simulink model "MovingAvg5"  (R2022a)
settings: Solver=FixedStepAuto  StartTime=0.0  StopTime=2500  FixedStep=1/3600  RelTol=1e-3
undefined symbols (not defined in the file or in its folder): dspblkCoreblockFVToolHelper, gcbh, sigbuilder_block
settings Model: SimulationMode=accelerator  Creator=rupak  LastModifiedBy=rupak
settings ConfigComp: DVTestSuiteOptimization=Auto  DVDefectChecker=off  DVDetectOutOfBounds=on  DVModelReferenceHarness=on  DVHarnessSource=Signal Editor

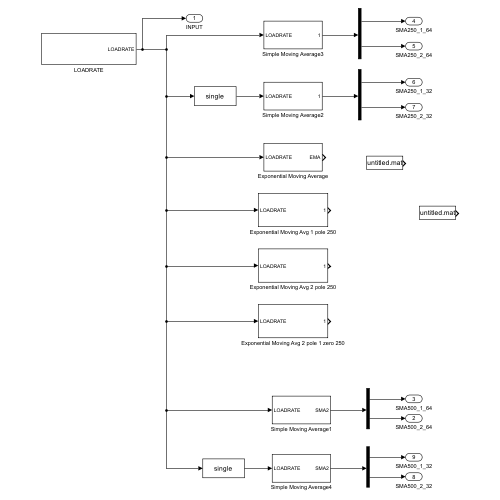
[thumbnail: Simulink's stored preview of the top-level diagram]
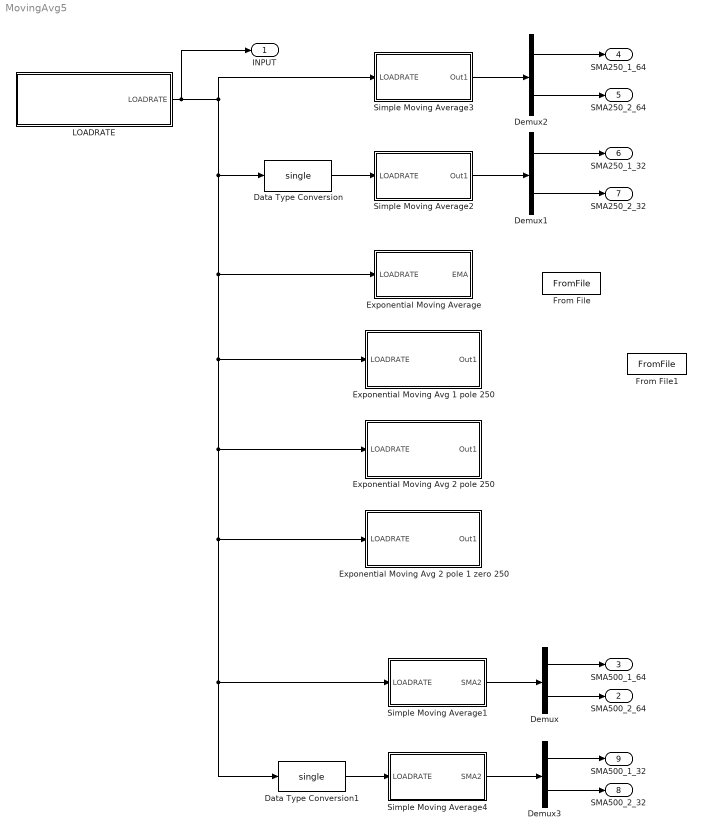
== system MovingAvg5 ==
  Data Type Conversion : DataTypeConversion  OutDataTypeStr=single  SaturateOnIntegerOverflow=off  RndMeth=Floor
  Data Type Conversion1 : DataTypeConversion  OutDataTypeStr=single  SaturateOnIntegerOverflow=off  RndMeth=Floor
  Demux{,1..3} (4 alike) : Demux  Outputs=2
  Exponential Moving Average : Subsystem
  Exponential Moving Avg 1 pole 250 : Subsystem
  Exponential Moving Avg 2 pole 1 zero 250 : Subsystem
  Exponential Moving Avg 2 pole 250 : Subsystem
  From File : FromFile  SampleTime=0
  From File1 : FromFile  SampleTime=0
  LOADRATE : Subsystem
  Simple Moving Average1 : Subsystem
  Simple Moving Average2 : Subsystem
  Simple Moving Average3 : Subsystem
  Simple Moving Average4 : Subsystem
  INPUT : Outport
  SMA500_2_64 : Outport  Port=2
  SMA500_1_64 : Outport  Port=3
  SMA250_1_64 : Outport  Port=4
  SMA250_2_64 : Outport  Port=5
  SMA250_1_32 : Outport  Port=6
  SMA250_2_32 : Outport  Port=7
  SMA500_2_32 : Outport  Port=8
  SMA500_1_32 : Outport  Port=9
  wires:
  Simple Moving Average1/1(SMA2) -> Demux/1
  Demux/1 -> SMA500_1_64/1
  Demux/2 -> SMA500_2_64/1
  Demux2/2 -> SMA250_2_64/1
  Demux2/1 -> SMA250_1_64/1
  Simple Moving Average3/1(Out1) -> Demux2/1
  LOADRATE/1(LOADRATE) -> Data Type Conversion/1, Exponential Moving Avg 1 pole 250/1(LOADRATE), Exponential Moving Avg 2 pole 250/1(LOADRATE), Exponential Moving Avg 2 pole 1 zero 250/1(LOADRATE), Simple Moving Average1/1(LOADRATE), Data Type Conversion1/1, Exponential Moving Average/1(LOADRATE), Simple Moving Average3/1(LOADRATE), INPUT/1
  Simple Moving Average2/1(Out1) -> Demux1/1
  Demux1/1 -> SMA250_1_32/1
  Demux1/2 -> SMA250_2_32/1
  Demux3/2 -> SMA500_2_32/1
  Demux3/1 -> SMA500_1_32/1
  Simple Moving Average4/1(SMA2) -> Demux3/1
  Data Type Conversion/1 -> Simple Moving Average2/1(LOADRATE)
  Data Type Conversion1/1 -> Simple Moving Average4/1(LOADRATE)

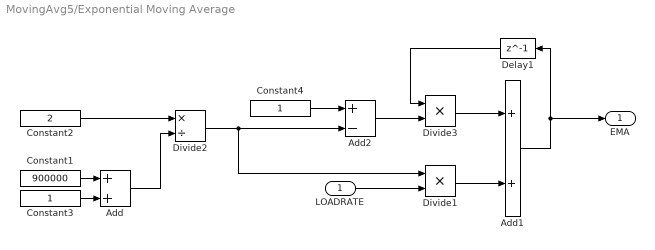
== system MovingAvg5/Exponential Moving Average ==
  LOADRATE : Inport
  Add : Sum
  Add1 : Sum
  Add2 : Sum  Inputs=+-
  Constant1 : Constant  Value=900000  OutDataTypeStr=single
  Constant2 : Constant  Value=2  OutDataTypeStr=single
  Constant3 : Constant  OutDataTypeStr=single
  Constant4 : Constant  OutDataTypeStr=single
  Delay1 : Delay  DelayLength=1  InitialCondition=60
  Divide1 : Product  Inputs=**
  Divide2 : Product  Inputs=*/
  Divide3 : Product  Inputs=**
  EMA : Outport
  wires:
  Add1/1 -> EMA/1, Delay1/1
  Divide1/1 -> Add1/2
  Constant2/1 -> Divide2/1
  Constant1/1 -> Add/1
  Constant3/1 -> Add/2
  Add/1 -> Divide2/2
  Delay1/1 -> Divide3/1
  Divide3/1 -> Add1/1
  Add2/1 -> Divide3/2
  Constant4/1 -> Add2/1
  Divide2/1 -> Add2/2, Divide1/1
  LOADRATE/1 -> Divide1/2

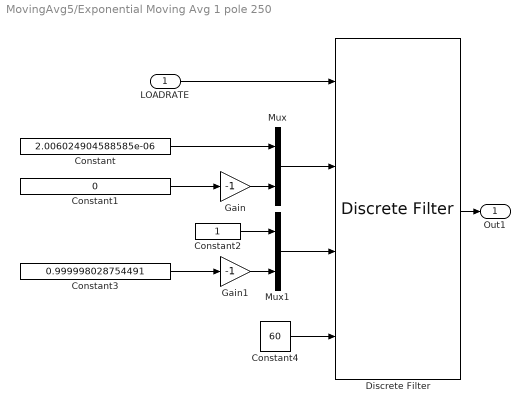
== system MovingAvg5/Exponential Moving Avg 1 pole 250 ==
  LOADRATE : Inport
  Constant : Constant  Value=2.006024904588585e-06
  Constant1 : Constant  Value=0
  Constant2 : Constant
  Constant3 : Constant  Value=0.999998028754491
  Constant4 : Constant  Value=60
  Discrete Filter : DiscreteFilter  LoadFcn=dspblkCoreblockFVToolHelper(gcbh,'load');  NumeratorSource=Input port  DenominatorSource=Input port  InitialStatesSource=Input port  FilterStructure=Direct form II transposed  a0EqualsOne=on
      settings: CopyFcn=dspblkCoreblockFVToolHelper(gcbh,'copy');  DeleteFcn=dspblkCoreblockFVToolHelper(gcbh,'close');  ModelCloseFcn=dspblkCoreblockFVToolHelper(gcbh,'close');  PreSaveFcn=dspblkCoreblockFVToolHelper(gcbh,'presave');  PostSaveFcn=dspblkCoreblockFVToolHelper(gcbh,'postsave');  CloseFcn=dspblkCoreblockFVToolHelper(gcbh,'close');  InputPortMap=u0,p1,p3,p5
  Gain : Gain  Gain=-1
  Gain1 : Gain  Gain=-1
  Mux : Mux  Inputs=2
  Mux1 : Mux  Inputs=2
  Out1 : Outport
  wires:
  Constant4/1 -> Discrete Filter/4
  Constant2/1 -> Mux1/1
  Constant3/1 -> Gain1/1
  Gain1/1 -> Mux1/2
  Mux/1 -> Discrete Filter/2
  Mux1/1 -> Discrete Filter/3
  Constant/1 -> Mux/1
  Constant1/1 -> Gain/1
  Gain/1 -> Mux/2
  LOADRATE/1 -> Discrete Filter/1
  Discrete Filter/1 -> Out1/1

== system MovingAvg5/Exponential Moving Avg 2 pole 1 zero 250 ==
  LOADRATE : Inport
  1st Filt : Subsystem
  2nd Filt : Subsystem
  Out1 : Outport
  wires:
  2nd Filt/1(Out1) -> Out1/1
  1st Filt/1(Out1) -> 2nd Filt/1(In1)
  LOADRATE/1 -> 1st Filt/1(In1)

== system MovingAvg5/Exponential Moving Avg 2 pole 250 ==
  LOADRATE : Inport
  1st Filt : Subsystem
  2nd Filt : Subsystem
  Out1 : Outport
  wires:
  LOADRATE/1 -> 1st Filt/1(In1)
  1st Filt/1(Out1) -> 2nd Filt/1(In1)
  2nd Filt/1(Out1) -> Out1/1

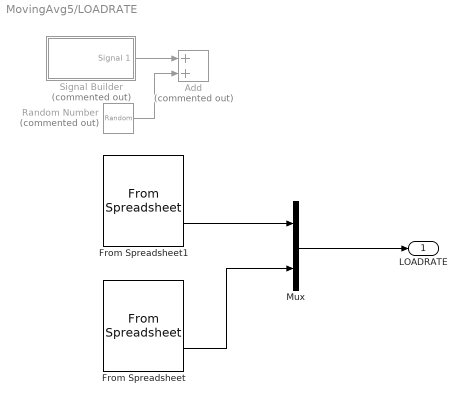
== system MovingAvg5/LOADRATE ==
  Add : Sum  Commented=on
  From Spreadsheet : FromSpreadsheet  FileName=C:\Users\rupak\OneDrive\Documents\MATLAB\Filter\Ransomes_NRTC-Full.xlsx  TreatFirstColumnAs=Data  SampleTime=1/3600
  From Spreadsheet1 : FromSpreadsheet  FileName=C:\Users\rupak\OneDrive\Documents\MATLAB\Filter\NRTC_3.xlsx  SheetName=NRTC_3  OutDataTypeStr=double  TreatFirstColumnAs=Data  SampleTime=1/3600
  Mux : Mux  Inputs=2
  Random Number : RandomNumber  Commented=on  Mean=5  SampleTime=1/3600
  Signal Builder : Subsystem  Tag=STV Subsys  Commented=on  LoadFcn=sigbuilder_block('load');  StartFcn=sigbuilder_block('start');  StopFcn=sigbuilder_block('stop');  ClipboardFcn=sigbuilder_block('clipboard');  mask(Sigbuilder block){tuvar=[0:10]}
      mask help: Simulink:masks:SigbuilderBlock_MD
      mask init:
      | if ~strcmp(get_param(bdroot(gcbh),'SimulationStatus'),'stopped') tuvar = sigbuilder_block('maskInit'); end
      settings: CopyFcn=sigbuilder_block('copy');  DeleteFcn=sigbuilder_block('delete');  ModelCloseFcn=sigbuilder_block('modelClose');  PreSaveFcn=sigbuilder_block('preSave');  PauseFcn=sigbuilder_block('pause');  ContinueFcn=sigbuilder_block('continue');  NameChangeFcn=sigbuilder_block('namechange');  OpenFcn=sigbuilder_block('open',[6 36 1428 675.75 ]);  CloseFcn=sigbuilder_block('close');
      mask Display: plot(0, 0, 100, 100,[2, 2, 32, 32, 2], [68, 8, 8, 68, 68],[32, 2], [38, 38], [32, 19, 2],[53, 60, 44], [32, 17, 17, 2],[16, 16, 31, 31]);txt = getActiveGroup(gcbh);text(2, 100, txt,'verticalAlignment', 'top');
  LOADRATE : Outport  SampleTime=1/3600  LockScale=on
  wires:
  Random Number/1 -> Add/2
  Signal Builder/1(Signal 1) -> Add/1
  Mux/1 -> LOADRATE/1
  From Spreadsheet/2 -> Mux/2
  From Spreadsheet1/2 -> Mux/1

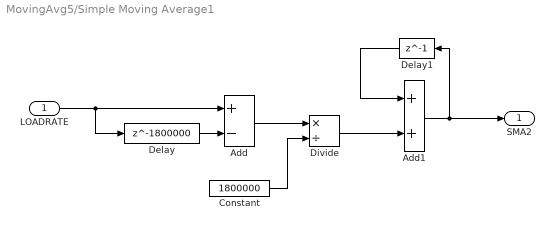
== system MovingAvg5/Simple Moving Average1 ==
  LOADRATE : Inport
  Add : Sum  Inputs=+-
  Add1 : Sum
  Constant : Constant  Value=1800000  OutDataTypeStr=single
  Delay : Delay  DelayLength=1800000  InitialCondition=60
  Delay1 : Delay  DelayLength=1  InitialCondition=60
  Divide : Product  Inputs=*/
  SMA2 : Outport
  wires:
  Divide/1 -> Add1/2
  Add1/1 -> Delay1/1, SMA2/1
  Add/1 -> Divide/1
  LOADRATE/1 -> Add/1, Delay/1
  Constant/1 -> Divide/2
  Delay1/1 -> Add1/1
  Delay/1 -> Add/2

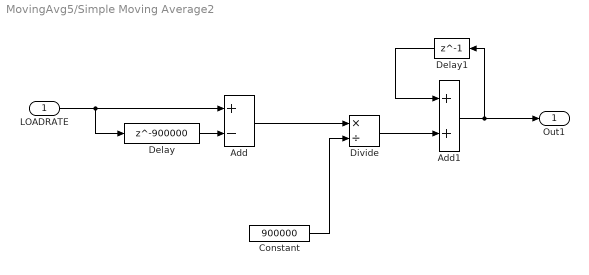
== system MovingAvg5/Simple Moving Average2 ==
  LOADRATE : Inport
  Add : Sum  Inputs=+-
  Add1 : Sum
  Constant : Constant  Value=900000  OutDataTypeStr=Inherit: Inherit via back propagation
  Delay : Delay  DelayLength=900000  InitialCondition=60
  Delay1 : Delay  DelayLength=1  InitialCondition=60
  Divide : Product  Inputs=*/
  Out1 : Outport
  wires:
  Add/1 -> Divide/1
  Delay/1 -> Add/2
  Delay1/1 -> Add1/1
  Constant/1 -> Divide/2
  LOADRATE/1 -> Delay/1, Add/1
  Add1/1 -> Out1/1, Delay1/1
  Divide/1 -> Add1/2

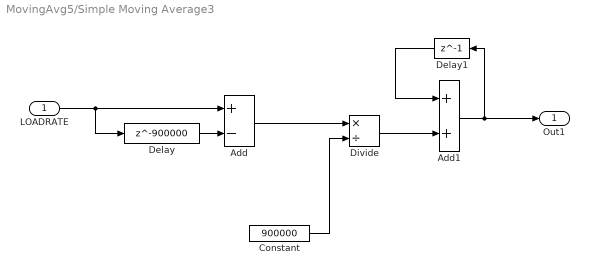
== system MovingAvg5/Simple Moving Average3 ==
  LOADRATE : Inport
  Add : Sum  Inputs=+-
  Add1 : Sum
  Constant : Constant  Value=900000  OutDataTypeStr=Inherit: Inherit via back propagation
  Delay : Delay  DelayLength=900000  InitialCondition=60
  Delay1 : Delay  DelayLength=1  InitialCondition=60
  Divide : Product  Inputs=*/
  Out1 : Outport
  wires:
  Divide/1 -> Add1/2
  Add1/1 -> Delay1/1, Out1/1
  LOADRATE/1 -> Add/1, Delay/1
  Constant/1 -> Divide/2
  Delay1/1 -> Add1/1
  Delay/1 -> Add/2
  Add/1 -> Divide/1

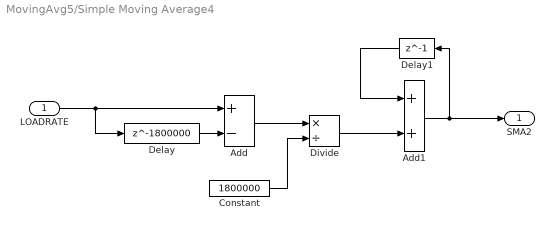
== system MovingAvg5/Simple Moving Average4 ==
  LOADRATE : Inport
  Add : Sum  Inputs=+-
  Add1 : Sum
  Constant : Constant  Value=1800000  OutDataTypeStr=single
  Delay : Delay  DelayLength=1800000  InitialCondition=60
  Delay1 : Delay  DelayLength=1  InitialCondition=60
  Divide : Product  Inputs=*/
  SMA2 : Outport
  wires:
  Delay/1 -> Add/2
  Delay1/1 -> Add1/1
  Constant/1 -> Divide/2
  LOADRATE/1 -> Delay/1, Add/1
  Add/1 -> Divide/1
  Add1/1 -> SMA2/1, Delay1/1
  Divide/1 -> Add1/2

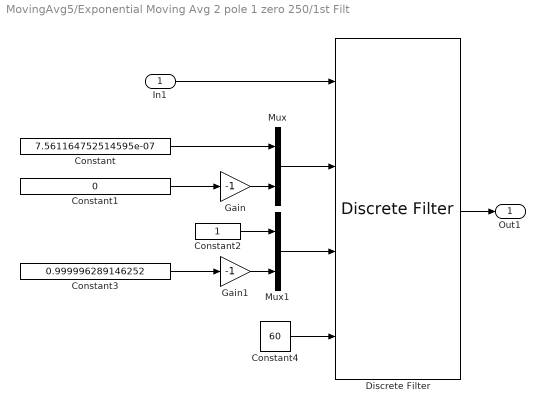
== system MovingAvg5/Exponential Moving Avg 2 pole 1 zero 250/1st Filt ==
  In1 : Inport
  Constant : Constant  Value=7.561164752514595e-07
  Constant1 : Constant  Value=0
  Constant2 : Constant
  Constant3 : Constant  Value=0.999996289146252
  Constant4 : Constant  Value=60
  Discrete Filter : DiscreteFilter  LoadFcn=dspblkCoreblockFVToolHelper(gcbh,'load');  NumeratorSource=Input port  DenominatorSource=Input port  InitialStatesSource=Input port  FilterStructure=Direct form II transposed  a0EqualsOne=on
      settings: CopyFcn=dspblkCoreblockFVToolHelper(gcbh,'copy');  DeleteFcn=dspblkCoreblockFVToolHelper(gcbh,'close');  ModelCloseFcn=dspblkCoreblockFVToolHelper(gcbh,'close');  PreSaveFcn=dspblkCoreblockFVToolHelper(gcbh,'presave');  PostSaveFcn=dspblkCoreblockFVToolHelper(gcbh,'postsave');  CloseFcn=dspblkCoreblockFVToolHelper(gcbh,'close');  InputPortMap=u0,p1,p3,p5
  Gain : Gain  Gain=-1
  Gain1 : Gain  Gain=-1
  Mux : Mux  Inputs=2
  Mux1 : Mux  Inputs=2
  Out1 : Outport
  wires:
  Discrete Filter/1 -> Out1/1
  Constant2/1 -> Mux1/1
  Constant3/1 -> Gain1/1
  Constant1/1 -> Gain/1
  Gain1/1 -> Mux1/2
  Constant4/1 -> Discrete Filter/4
  Constant/1 -> Mux/1
  Gain/1 -> Mux/2
  In1/1 -> Discrete Filter/1
  Mux1/1 -> Discrete Filter/3
  Mux/1 -> Discrete Filter/2

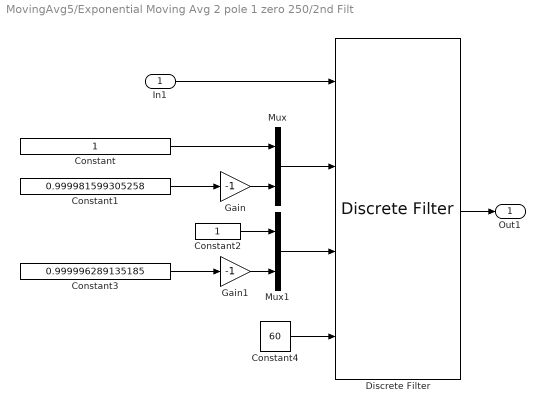
== system MovingAvg5/Exponential Moving Avg 2 pole 1 zero 250/2nd Filt ==
  In1 : Inport
  Constant : Constant
  Constant1 : Constant  Value=0.999981599305258
  Constant2 : Constant
  Constant3 : Constant  Value=0.999996289135185
  Constant4 : Constant  Value=60
  Discrete Filter : DiscreteFilter  LoadFcn=dspblkCoreblockFVToolHelper(gcbh,'load');  NumeratorSource=Input port  DenominatorSource=Input port  InitialStatesSource=Input port  FilterStructure=Direct form II transposed  a0EqualsOne=on
      settings: CopyFcn=dspblkCoreblockFVToolHelper(gcbh,'copy');  DeleteFcn=dspblkCoreblockFVToolHelper(gcbh,'close');  ModelCloseFcn=dspblkCoreblockFVToolHelper(gcbh,'close');  PreSaveFcn=dspblkCoreblockFVToolHelper(gcbh,'presave');  PostSaveFcn=dspblkCoreblockFVToolHelper(gcbh,'postsave');  CloseFcn=dspblkCoreblockFVToolHelper(gcbh,'close');  InputPortMap=u0,p1,p3,p5
  Gain : Gain  Gain=-1
  Gain1 : Gain  Gain=-1
  Mux : Mux  Inputs=2
  Mux1 : Mux  Inputs=2
  Out1 : Outport
  wires:
  Mux/1 -> Discrete Filter/2
  Mux1/1 -> Discrete Filter/3
  In1/1 -> Discrete Filter/1
  Gain/1 -> Mux/2
  Constant/1 -> Mux/1
  Constant4/1 -> Discrete Filter/4
  Gain1/1 -> Mux1/2
  Constant1/1 -> Gain/1
  Constant3/1 -> Gain1/1
  Constant2/1 -> Mux1/1
  Discrete Filter/1 -> Out1/1

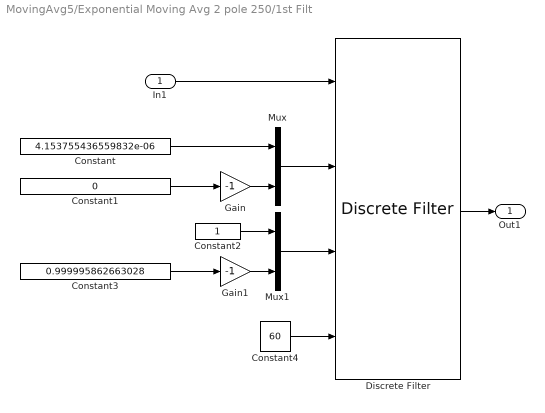
== system MovingAvg5/Exponential Moving Avg 2 pole 250/1st Filt ==
  In1 : Inport
  Constant : Constant  Value=4.153755436559832e-06
  Constant1 : Constant  Value=0
  Constant2 : Constant
  Constant3 : Constant  Value=0.999995862663028
  Constant4 : Constant  Value=60
  Discrete Filter : DiscreteFilter  LoadFcn=dspblkCoreblockFVToolHelper(gcbh,'load');  NumeratorSource=Input port  DenominatorSource=Input port  InitialStatesSource=Input port  FilterStructure=Direct form II transposed  a0EqualsOne=on
      settings: CopyFcn=dspblkCoreblockFVToolHelper(gcbh,'copy');  DeleteFcn=dspblkCoreblockFVToolHelper(gcbh,'close');  ModelCloseFcn=dspblkCoreblockFVToolHelper(gcbh,'close');  PreSaveFcn=dspblkCoreblockFVToolHelper(gcbh,'presave');  PostSaveFcn=dspblkCoreblockFVToolHelper(gcbh,'postsave');  CloseFcn=dspblkCoreblockFVToolHelper(gcbh,'close');  InputPortMap=u0,p1,p3,p5
  Gain : Gain  Gain=-1
  Gain1 : Gain  Gain=-1
  Mux : Mux  Inputs=2
  Mux1 : Mux  Inputs=2
  Out1 : Outport
  wires:
  Mux/1 -> Discrete Filter/2
  Mux1/1 -> Discrete Filter/3
  In1/1 -> Discrete Filter/1
  Gain/1 -> Mux/2
  Constant/1 -> Mux/1
  Constant4/1 -> Discrete Filter/4
  Gain1/1 -> Mux1/2
  Constant1/1 -> Gain/1
  Constant3/1 -> Gain1/1
  Constant2/1 -> Mux1/1
  Discrete Filter/1 -> Out1/1

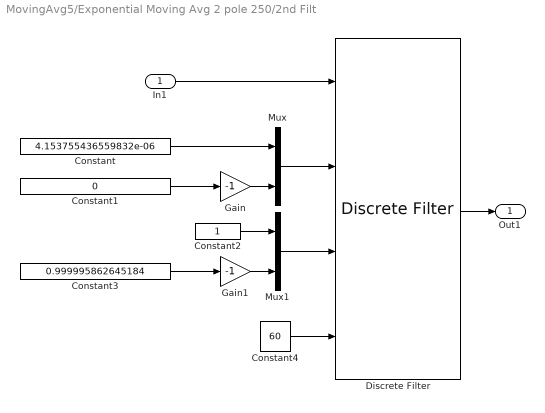
== system MovingAvg5/Exponential Moving Avg 2 pole 250/2nd Filt ==
  In1 : Inport
  Constant : Constant  Value=4.153755436559832e-06
  Constant1 : Constant  Value=0
  Constant2 : Constant
  Constant3 : Constant  Value=0.999995862645184
  Constant4 : Constant  Value=60
  Discrete Filter : DiscreteFilter  LoadFcn=dspblkCoreblockFVToolHelper(gcbh,'load');  NumeratorSource=Input port  DenominatorSource=Input port  InitialStatesSource=Input port  FilterStructure=Direct form II transposed  a0EqualsOne=on
      settings: CopyFcn=dspblkCoreblockFVToolHelper(gcbh,'copy');  DeleteFcn=dspblkCoreblockFVToolHelper(gcbh,'close');  ModelCloseFcn=dspblkCoreblockFVToolHelper(gcbh,'close');  PreSaveFcn=dspblkCoreblockFVToolHelper(gcbh,'presave');  PostSaveFcn=dspblkCoreblockFVToolHelper(gcbh,'postsave');  CloseFcn=dspblkCoreblockFVToolHelper(gcbh,'close');  InputPortMap=u0,p1,p3,p5
  Gain : Gain  Gain=-1
  Gain1 : Gain  Gain=-1
  Mux : Mux  Inputs=2
  Mux1 : Mux  Inputs=2
  Out1 : Outport
  wires:
  Discrete Filter/1 -> Out1/1
  Constant2/1 -> Mux1/1
  Constant3/1 -> Gain1/1
  Constant1/1 -> Gain/1
  Gain1/1 -> Mux1/2
  Constant4/1 -> Discrete Filter/4
  Constant/1 -> Mux/1
  Gain/1 -> Mux/2
  In1/1 -> Discrete Filter/1
  Mux1/1 -> Discrete Filter/3
  Mux/1 -> Discrete Filter/2

== system MovingAvg5/LOADRATE/Signal Builder ==
  Demux : Demux  Tag=STV Demux  Outputs=1
      settings: DisplayOption=none
  FromWs : FromWorkspace  Tag=STV FromWs  VariableName=tuvar
      SigBuilderData=|
      | common.afterFinalStr = 'Extrapolate'
      | common.sampleTime = 0
      | dataSet.timeRange = [0 1500]
      | dataSet.name = 'Group 1'
      | sbobj.Groups.Name = 'Group 1'
      | sbobj.Groups.Signals.Name = 'Signal 1'
      | sbobj.Groups.Signals.XData = [0 4 4 10 12 16 18 20 24 30 36 40 44 50 56 60 60 64 64 70 74 78 80 82 86 88 88 90 92 98 104 108 112 118 122 128 132 138 144 150 154 158 160 162 166 170 174 176 180 182 184 190 196 200 202 208 216 226 232 240 250 260 266 278 284 292 296 300 304 310 316 322 326 338 346 356 362 368 374 378 384 392 400 406 414 420 424 430 432 438 442 446 450 458 464 470 476 482 487 489 490 496 500 508 518 528 536 546 552 558 562 570 582 588 592 598 606 620 626 634 644 650 664 673 674 682 696 706 716 724 734 744 756 764 772 780 790 800 808 816 826 834 844 856 864 872 880 890 904 914 928 942 952 960 972 994 1072 1116 1126 1134 1142 1156 1160 1166 1176 1182 1190 1198 1208 1220 1228 1235 1246 1258 1265 1277 1287 1297 1308 1323 1332 1342 1347 1355 1361 1371 1379 1389 1402 1408 1415 1422 1435 1439 1446 1453 1469 1475 1485 1492 1495 1500]
      | sbobj.Groups.Signals.YData = [2 96.2 69.2 84 75 56.8 90 74.4 80.8 65.2 91 85.4 67.4 77.4 55.6 61 48 18.6 31.6 51.4 51.4 38.4 56.4 63.4 86.6 78.2 83.2 71 57.6 78.6 36 85.4 57 39 41 43.8 57 45.6 42.8 53 78.2 68.4 74 67 56.6 61 55.6 34 51.4 74.2 50.8 93 74.4 78 61.2 52 58 40.6 58 54.4 42.6 71 47.8 56 50.8 69 48.2 70 54.8 48.2 54.6 34.4 46.4 55.6 42.6 57.2 33.2 85.8 53.6 59 54.6 49.4 63 54.8 76.4 57.2 70 64.8 35.4 64.2 51.8 57 47.2 59.8 52.6 69 53.4 70 64.8 61.4 45.4 53.4 32 46.8 42.6 45 39.8 53.6 50.2 59.2 56.8 55 62.2 53.6 56 58.8 56 63 55 66 59.6 71 67.8 70.8 63.4 58 63.2 60.2 63 74.8 63.8 68 59.8 65.6 55.6 63.2 62.2 68.6 65.6 69.6 69 75.2 70 72 66.6 63.4 86 74.4 83.4 79 61.6 69.8 51.2 60.4 40.4 49.6 33 40.6 45.8 43.4 49.8 45 48.8 55 49.6 44.4 56 52 67 55 52 56.6 48.6 57 52.4 62.2 46.8 59.2 60.6 57.4 65.2 63.2238095238 66.2 76.2 70 75 82.2 72.2 75.4 69.4 72.4 65.2 66.2 64.0953846154 65.6 65.4 65.4 59.8 59.6 63.2 57.2 51.4]
      | sbobj.Groups.TimeRange = [0 1500]
  Signal 1 : Outport  Tag=STV Outport
  wires:
  Demux/1 -> Signal 1/1
  FromWs/1 -> Demux/1
